simulink model "Lombardini_dual_fuel"  (R2024b)
settings: Solver=FixedStepAuto  StartTime=0.0  StopTime=2000  RelTol=1e-3  EnableMultiTasking=on
PreLoadFcn:
  | try, eval([bdroot '_setup']); catch, eval('model_setup', ''); end
InitFcn:
  | try, eval([bdroot '_setup']); catch, eval('model_setup', ''); end
model workspace (MAT data in the model file):
  PID_rpm = [1000 2000 3000 4000]
undefined symbols (not defined in the file): ECU555, motohawk_build_version, motohawk_get_target_image, motohawk_target_type, motohawk_trunc_name, motohawk_vardec_path
libraries: MotoHawk_lib x118, motohawk_annotations_lib x23, dspstat3 x13, motohawk_examples_lib x1, MotoHawk_Protocols_lib x1
(part 2 of 5)

== system Lombardini_dual_fuel/Background ==
  FMU : Inport
  f : TriggerPort  TriggerType=function-call  VariantControl=Variant
  Plant : Subsystem  mask(Display Image File){image_file='engine.jpg'}
      mask prompts: image_file "Image File"
      mask help:
      | Enter an image file on the current MATLAB path to display on this block.
      |
      | Double-clicking this block opens the contents of the subsystem.  Right-click and select 'Mask parameters...' to select a new image file.
      |
      | To use just the mask of this block in a model, but supply your own contents, break the link to the library.
      mask init:
      | try,
      | 	img = imread(image_file);
      | 	motohawk_block_image(gcb, image_file);
      | catch,
      | 	img = imread('image_not_found.jpg');
      | end
      settings: OpenFcn=open_system(gcb,'force')  MoveFcn=motohawk_block_image(gcb, motohawk_get_param_ws(gcb, 'image_file'));
      mask Display: image(img);
  motohawk_TitleBlock : motohawk_annotations_lib/motohawk_TitleBlock  BlockType_='Mototron_Title_Block'  ttl=[strrep(get_param(bdroot, 'Description') , '_', '\_') '\newline\rm' get_param(gcs, 'Name')]  copyright="'THE INFORMATION CONTAINED IN THIS\\newlineDRAWING IS THE SOLE PROPERTY OF\\newlineWOODWARD.  ANY REPRODUCTION IN\\newline PART OR AS A WHOLE WITHOUT THE\\newlineWRITTEN PERMISSION OF WOODWARD\\newline IS PROHIBITED.\\fontsize{16}\\rm\\copyright\\rm\\fontsize{10} 2017'"  address='\fontsize{22}\it\fontname{Arial Black}Woodward \fontname{Arial}\fontsize{10}\newline1081 Woodward Way, Fort Collins, CO, 80524\newlinemcs.woodward.com'  image_file='mh.jpg'  pretty_print=on  edit_text=[strrep(get_param(bdroot, 'Description') , '_', '\_') '\newline\rm' get_param(gcs, 'Name')]  edit_as=5
      settings: SourceProductName=MotoHawk Annotations
  motohawk_code_coverage : MotoHawk_lib/Extra Development Blocks/motohawk_code_coverage
      settings: SourceProductName=MotoHawk
  wires:
  FMU/1 -> Plant/1(FMU)

== system Lombardini_dual_fuel/Foreground ==
  FMU : Inport
  f : TriggerPort  TriggerType=function-call  VariantControl=Variant
  Controller : Subsystem  mask(Display Image File){image_file=motohawk_get_target_image(motohawk_target_type(bdroot))}
      mask prompts: image_file "Image File"
      mask help:
      | Enter an image file on the current MATLAB path to display on this block.
      |
      | Double-clicking this block opens the contents of the subsystem.  Right-click and select 'Mask parameters...' to select a new image file.
      |
      | To use just the mask of this block in a model, but supply your own contents, break the link to the library.
      mask init:
      | try,
      | 	img = imread(image_file);
      | 	motohawk_block_image(gcb, image_file);
      | catch,
      | 	img = imread('image_not_found.jpg');
      | end
      settings: OpenFcn=open_system(gcb,'force')  MoveFcn=motohawk_block_image(gcb, motohawk_get_param_ws(gcb, 'image_file'));
      mask Display: image(img);
  Plant : Subsystem  mask(Display Image File){image_file='engine.jpg'}
      mask prompts: image_file "Image File"
      mask help:
      | Enter an image file on the current MATLAB path to display on this block.
      |
      | Double-clicking this block opens the contents of the subsystem.  Right-click and select 'Mask parameters...' to select a new image file.
      |
      | To use just the mask of this block in a model, but supply your own contents, break the link to the library.
      mask init:
      | try,
      | 	img = imread(image_file);
      | 	motohawk_block_image(gcb, image_file);
      | catch,
      | 	img = imread('image_not_found.jpg');
      | end
      settings: OpenFcn=open_system(gcb,'force')  MoveFcn=motohawk_block_image(gcb, motohawk_get_param_ws(gcb, 'image_file'));
      mask Display: image(img);
  motohawk_TitleBlock : motohawk_annotations_lib/motohawk_TitleBlock  BlockType_='Mototron_Title_Block'  ttl=[strrep(get_param(bdroot, 'Description') , '_', '\_') '\newline\rm' get_param(gcs, 'Name')]  copyright="'THE INFORMATION CONTAINED IN THIS\\newlineDRAWING IS THE SOLE PROPERTY OF\\newlineWOODWARD.  ANY REPRODUCTION IN\\newline PART OR AS A WHOLE WITHOUT THE\\newlineWRITTEN PERMISSION OF WOODWARD\\newline IS PROHIBITED.\\fontsize{16}\\rm\\copyright\\rm\\fontsize{10} 2017'"  address='\fontsize{22}\it\fontname{Arial Black}Woodward \fontname{Arial}\fontsize{10}\newline1081 Woodward Way, Fort Collins, CO, 80524\newlinemcs.woodward.com'  image_file='mh.jpg'  pretty_print=on  edit_text=[strrep(get_param(bdroot, 'Description') , '_', '\_') '\newline\rm' get_param(gcs, 'Name')]  edit_as=5
      settings: SourceProductName=MotoHawk Annotations
  motohawk_code_coverage : MotoHawk_lib/Extra Development Blocks/motohawk_code_coverage
      settings: SourceProductName=MotoHawk
  Out1 : Outport
  wires:
  Plant/1(SensorBus) -> Controller/1(Sensors)
  Controller/1(Actuators) -> Out1/1, Plant/1(ActuatorBus)
  FMU/1 -> Plant/2(FMU)

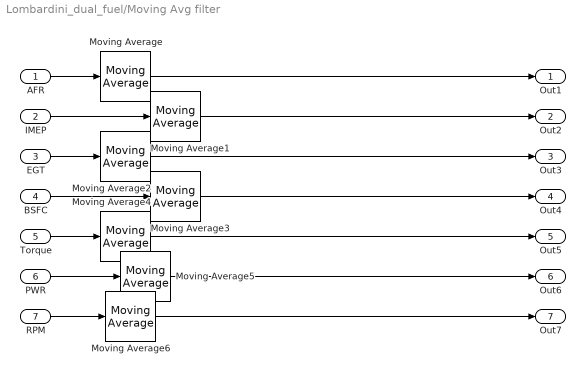
== system Lombardini_dual_fuel/Moving Avg filter ==
  AFR : Inport
  IMEP : Inport  Port=2
  EGT : Inport  Port=3
  BSFC : Inport  Port=4
  Torque : Inport  Port=5
  PWR : Inport  Port=6
  RPM : Inport  Port=7
  Moving Average : dspstat3/Moving Average  Method=Sliding window  ForgettingFactorPort=off  SpecifyWindowLength=on  WindowLength=200  OverlapLength=199  AllowArbitraryInputLength=off  ForgettingFactor=0.9  SimulateUsing=Interpreted execution
  Moving Average{1..6} (6 alike) : dspstat3/Moving Average  Method=Sliding window  ForgettingFactorPort=off  SpecifyWindowLength=on  WindowLength=100  OverlapLength=99  AllowArbitraryInputLength=off  ForgettingFactor=0.9  SimulateUsing=Interpreted execution
  Out1 : Outport
  Out2 : Outport  Port=2
  Out3 : Outport  Port=3
  Out4 : Outport  Port=4
  Out5 : Outport  Port=5
  Out6 : Outport  Port=6
  Out7 : Outport  Port=7
  wires:
  AFR/1 -> Moving Average/1
  RPM/1 -> Moving Average6/1
  IMEP/1 -> Moving Average1/1
  Moving Average1/1 -> Out2/1
  Moving Average2/1 -> Out3/1
  Moving Average5/1 -> Out6/1
  Moving Average/1 -> Out1/1
  BSFC/1 -> Moving Average3/1
  Moving Average4/1 -> Out5/1
  Torque/1 -> Moving Average4/1
  PWR/1 -> Moving Average5/1
  Moving Average3/1 -> Out4/1
  EGT/1 -> Moving Average2/1
  Moving Average6/1 -> Out7/1

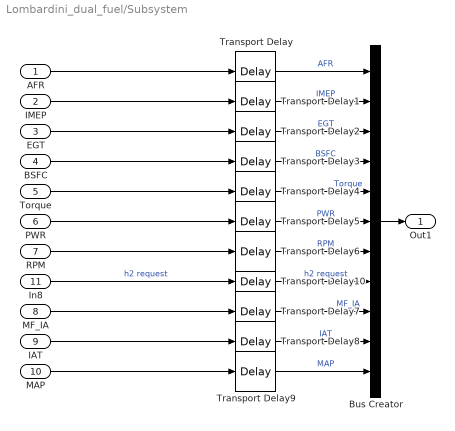
== system Lombardini_dual_fuel/Subsystem ==
  AFR : Inport
  IMEP : Inport  Port=2
  EGT : Inport  Port=3
  BSFC : Inport  Port=4
  Torque : Inport  Port=5
  PWR : Inport  Port=6
  RPM : Inport  Port=7
  MF_IA : Inport  Port=8
  IAT : Inport  Port=9
  MAP : Inport  Port=10
  In8 : Inport  Port=11
  Bus Creator : BusCreator  Inputs=11
  Transport Delay{,1..10} (11 alike) : TransportDelay  DelayTime=0.1
  Out1 : Outport
  wires:
  Transport Delay6/1 -> Bus Creator/7  "RPM"
  Transport Delay1/1 -> Bus Creator/2  "IMEP"
  Transport Delay5/1 -> Bus Creator/6  "PWR"
  Transport Delay2/1 -> Bus Creator/3  "EGT"
  AFR/1 -> Transport Delay/1
  Transport Delay/1 -> Bus Creator/1  "AFR"
  Transport Delay3/1 -> Bus Creator/4  "BSFC"
  Transport Delay4/1 -> Bus Creator/5  "Torque"
  RPM/1 -> Transport Delay6/1
  IMEP/1 -> Transport Delay1/1
  EGT/1 -> Transport Delay2/1
  PWR/1 -> Transport Delay5/1
  Bus Creator/1 -> Out1/1
  Torque/1 -> Transport Delay4/1
  BSFC/1 -> Transport Delay3/1
  In8/1 -> Transport Delay10/1  "h2 request"
  MF_IA/1 -> Transport Delay7/1
  Transport Delay7/1 -> Bus Creator/9  "MF_IA"
  MAP/1 -> Transport Delay9/1
  IAT/1 -> Transport Delay8/1
  Transport Delay8/1 -> Bus Creator/10  "IAT"
  Transport Delay9/1 -> Bus Creator/11  "MAP"
  Transport Delay10/1 -> Bus Creator/8  "h2 request"

== system Lombardini_dual_fuel/Subsystem1 ==
  In1 : Inport
  In3 : Inport  Port=2
  Moving Average1 : dspstat3/Moving Average  Method=Sliding window  ForgettingFactorPort=off  SpecifyWindowLength=on  WindowLength=100  OverlapLength=99  AllowArbitraryInputLength=off  ForgettingFactor=0.9  SimulateUsing=Interpreted execution
  Moving Average4 : dspstat3/Moving Average  Method=Sliding window  ForgettingFactorPort=off  SpecifyWindowLength=on  WindowLength=100  OverlapLength=99  AllowArbitraryInputLength=off  ForgettingFactor=0.9  SimulateUsing=Interpreted execution
  fuel energy : Outport
  imep gas exchange : Outport  Port=2
  wires:
  Moving Average1/1 -> imep gas exchange/1  "imep gas exchange"
  In1/1 -> Moving Average4/1
  In3/1 -> Moving Average1/1
  Moving Average4/1 -> fuel energy/1  "fuel energy"

== system Lombardini_dual_fuel/Background/Plant ==
  FMU : Inport
  Sensors : Subsystem
  motohawk_TitleBlock : motohawk_annotations_lib/motohawk_TitleBlock  BlockType_='Mototron_Title_Block'  ttl=[get_param(bdroot, 'Description') '\rm\newlineRead H/W sensors and Drive H/W actuators\newlineThe Sensors and Actuators busses should contain signals in engineering units\newline']  copyright="'THE INFORMATION CONTAINED IN THIS\\newlineDRAWING IS THE SOLE PROPERTY OF\\newlineWOODWARD.  ANY REPRODUCTION IN\\newline PART OR AS A WHOLE WITHOUT THE\\newlineWRITTEN PERMISSION OF WOODWARD\\newline IS PROHIBITED.\\fontsize{16}\\rm\\copyright\\rm\\fontsize{10} 2017'"  address='\fontsize{22}\it\fontname{Arial Black}Woodward \fontname{Arial}\fontsize{10}\newline1081 Woodward Way, Fort Collins, CO, 80524\newlinemcs.woodward.com'  image_file='mh.jpg'  pretty_print=on  edit_text=|  edit_as=6
      | [get_param(bdroot, 'Description') '\rm
      | 
      | 
      | Read H/W sensors and Drive H/W actuators
      | 
      | 
      | The Sensors and Actuators busses should contain signals in engineering units
      | 
      | 
      | ']
      settings: SourceProductName=MotoHawk Annotations
  wires:
  FMU/1 -> Sensors/1(In1)

== system Lombardini_dual_fuel/Foreground/Controller ==
  Sensors : Inport
  Calibration : Subsystem
  Characterization : Subsystem
  Controller : Subsystem
  Virtual Sensors : Subsystem
  motohawk_TitleBlock : motohawk_annotations_lib/motohawk_TitleBlock  BlockType_='Mototron_Title_Block'  ttl=[get_param(bdroot, 'Description') '\rm\newlineTop-level design of Controller\newlineVirtual Sensors model signals that are not available as H/W sensors\newlineCharacterization converts or linearizes Controller units to actuator units\newline']  copyright="'THE INFORMATION CONTAINED IN THIS\\newlineDRAWING IS THE SOLE PROPERTY OF\\newlineWOODWARD.  ANY REPRODUCTION IN\\newline PART OR AS A WHOLE WITHOUT THE\\newlineWRITTEN PERMISSION OF WOODWARD\\newline IS PROHIBITED.\\fontsize{16}\\rm\\copyright\\rm\\fontsize{10} 2017'"  address='\fontsize{22}\it\fontname{Arial Black}Woodward \fontname{Arial}\fontsize{10}\newline1081 Woodward Way, Fort Collins, CO, 80524\newlinemcs.woodward.com'  image_file='mh.jpg'  pretty_print=on  edit_text=|  edit_as=6
      | [get_param(bdroot, 'Description') '\rm
      | 
      | 
      | Top-level design of Controller
      | 
      | 
      | Virtual Sensors model signals that are not available as H/W sensors
      | 
      | 
      | Characterization converts or linearizes Controller units to actuator units
      | 
      | 
      | ']
      settings: SourceProductName=MotoHawk Annotations
  Actuators : Outport  VectorParamsAs1DForOutWhenUnconnected=off
  wires:
  Controller/1(Actuators) -> Characterization/1(Control)
  Virtual Sensors/1(Synth) -> Calibration/1(Sensor data), Controller/1(Sensors)
  Sensors/1 -> Virtual Sensors/1(Real)
  Characterization/1(Actuators) -> Actuators/1
  Calibration/1(Calibration data) -> Controller/2(Calibration)

== system Lombardini_dual_fuel/Foreground/Plant ==
  ActuatorBus : Inport
  FMU : Inport  Port=2
  Actuators : Subsystem
  Sensors : Subsystem
  motohawk_TitleBlock : motohawk_annotations_lib/motohawk_TitleBlock  BlockType_='Mototron_Title_Block'  ttl=[get_param(bdroot, 'Description') '\rm\newlineRead H/W sensors and Drive H/W actuators\newlineThe Sensors and Actuators busses should contain signals in engineering units\newline']  copyright="'THE INFORMATION CONTAINED IN THIS\\newlineDRAWING IS THE SOLE PROPERTY OF\\newlineWOODWARD.  ANY REPRODUCTION IN\\newline PART OR AS A WHOLE WITHOUT THE\\newlineWRITTEN PERMISSION OF WOODWARD\\newline IS PROHIBITED.\\fontsize{16}\\rm\\copyright\\rm\\fontsize{10} 2017'"  address='\fontsize{22}\it\fontname{Arial Black}Woodward \fontname{Arial}\fontsize{10}\newline1081 Woodward Way, Fort Collins, CO, 80524\newlinemcs.woodward.com'  image_file='mh.jpg'  pretty_print=on  edit_text=|  edit_as=6
      | [get_param(bdroot, 'Description') '\rm
      | 
      | 
      | Read H/W sensors and Drive H/W actuators
      | 
      | 
      | The Sensors and Actuators busses should contain signals in engineering units
      | 
      | 
      | ']
      settings: SourceProductName=MotoHawk Annotations
  SensorBus : Outport  VectorParamsAs1DForOutWhenUnconnected=off
  wires:
  Sensors/1(Sensors) -> SensorBus/1
  ActuatorBus/1 -> Actuators/1(Actuators)
  FMU/1 -> Sensors/1(In1)

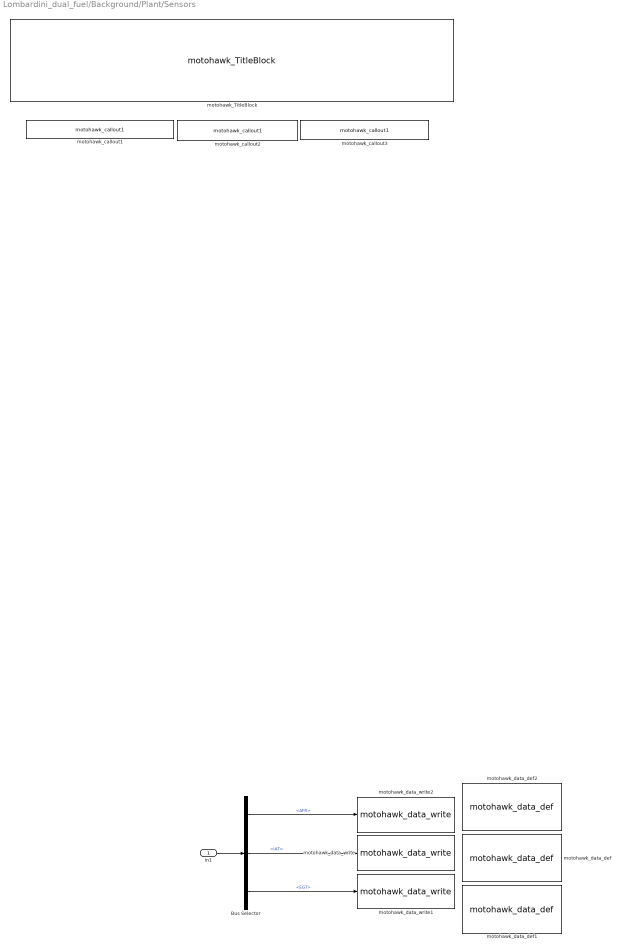
== system Lombardini_dual_fuel/Background/Plant/Sensors ==
  In1 : Inport
  Bus Selector : BusSelector  OutputSignals=AFR,IAT,EGT
  motohawk_TitleBlock : motohawk_annotations_lib/motohawk_TitleBlock  BlockType_='Mototron_Title_Block'  ttl=[get_param(bdroot, 'Description') '\rm\newlineSample H/W sensors, such as:\newlineA/D converters, digital inputs, frequency inputs, and engine encoder\newline']  copyright="'THE INFORMATION CONTAINED IN THIS\\newlineDRAWING IS THE SOLE PROPERTY OF\\newlineWOODWARD.  ANY REPRODUCTION IN\\newline PART OR AS A WHOLE WITHOUT THE\\newlineWRITTEN PERMISSION OF WOODWARD\\newline IS PROHIBITED.\\fontsize{16}\\rm\\copyright\\rm\\fontsize{10} 2017'"  address='\fontsize{22}\it\fontname{Arial Black}Woodward \fontname{Arial}\fontsize{10}\newline1081 Woodward Way, Fort Collins, CO, 80524\newlinemcs.woodward.com'  image_file='mh.jpg'  pretty_print=on  edit_text=|  edit_as=6
      | [get_param(bdroot, 'Description') '\rm
      | 
      | 
      | Sample H/W sensors, such as:
      | 
      | 
      | A/D converters, digital inputs, frequency inputs, and engine encoder
      | 
      | 
      | ']
      settings: SourceProductName=MotoHawk Annotations
  motohawk_callout1 : motohawk_annotations_lib/motohawk_callout1  BlockType_='Mototron_harea'  desc='Read from H/W'  edit_text=Read from H/W  edit_as=0
      settings: SourceProductName=MotoHawk Annotations
  motohawk_callout2 : motohawk_annotations_lib/motohawk_callout1  BlockType_='Mototron_harea'  desc='Convert to Engineering Units'  edit_text=Convert to Engineering Units  edit_as=0
      settings: SourceProductName=MotoHawk Annotations
  motohawk_callout3 : motohawk_annotations_lib/motohawk_callout1  BlockType_='Mototron_harea'  desc='Create a Bus of Sensors'  edit_text=Create a Bus of Sensors  edit_as=0
      settings: SourceProductName=MotoHawk Annotations
  motohawk_data_def : MotoHawk_lib/Data Storage Blocks/motohawk_data_def  nam='IAT_slow'  container_nam=''  data=5  typ=double  struct_nam='MyStruct'  storage=Volatile  outputRef=off  mem_region_use=off  mem_region_name='SERIAL_EE'  use_vardec=on  window=Display  ovr_cals=on  read_level=1  write_level=1  view_as=Number  enum_struct={'Disabled', 'Enabled'}  vector_style=Wide Row  row_header_enum=''  col_header_enum=''  mototune_group=motohawk_vardec_path(gcb)  help=''  units=''  min_val=-inf  max_val=inf  precision=''  gain=1  offset=0  exp=1  use_help_units=off  use_header_enum=off  use_min_max=off  use_precision=off  use_mototune_group=off  eval_name=MyData  struct_instances=motohawk_sfun_data_def_struct_instances  vardecs=motohawk_sfun_data_def_vardecs  data_stores=motohawk_sfun_data_def_data_stores
      settings: SourceProductName=MotoHawk
  motohawk_data_def1 : MotoHawk_lib/Data Storage Blocks/motohawk_data_def  nam='EGT_100ms'  container_nam=''  data=5  typ=double  struct_nam='MyStruct'  storage=Volatile  outputRef=off  mem_region_use=off  mem_region_name='SERIAL_EE'  use_vardec=on  window=Display  ovr_cals=on  read_level=1  write_level=1  view_as=Number  enum_struct={'Disabled', 'Enabled'}  vector_style=Wide Row  row_header_enum=''  col_header_enum=''  mototune_group=motohawk_vardec_path(gcb)  help=''  units=''  min_val=-inf  max_val=inf  precision=''  gain=1  offset=0  exp=1  use_help_units=off  use_header_enum=off  use_min_max=off  use_precision=off  use_mototune_group=off  eval_name=MyData  struct_instances=motohawk_sfun_data_def_struct_instances  vardecs=motohawk_sfun_data_def_vardecs  data_stores=motohawk_sfun_data_def_data_stores
      settings: SourceProductName=MotoHawk
  motohawk_data_def2 : MotoHawk_lib/Data Storage Blocks/motohawk_data_def  nam='AFR_100ms'  container_nam=''  data=5  typ=double  struct_nam='MyStruct'  storage=Volatile  outputRef=off  mem_region_use=off  mem_region_name='SERIAL_EE'  use_vardec=on  window=Display  ovr_cals=on  read_level=1  write_level=1  view_as=Number  enum_struct={'Disabled', 'Enabled'}  vector_style=Wide Row  row_header_enum=''  col_header_enum=''  mototune_group=motohawk_vardec_path(gcb)  help=''  units=''  min_val=-inf  max_val=inf  precision=''  gain=1  offset=0  exp=1  use_help_units=off  use_header_enum=off  use_min_max=off  use_precision=off  use_mototune_group=off  eval_name=MyData  struct_instances=motohawk_sfun_data_def_struct_instances  vardecs=motohawk_sfun_data_def_vardecs  data_stores=motohawk_sfun_data_def_data_stores
      settings: SourceProductName=MotoHawk
  motohawk_data_write : MotoHawk_lib/Data Storage Blocks/motohawk_data_write  source=Lookup By Name  structure=Scalar  operation=Write entire data structure at once  sz_vec=9  sz_row=2  sz_col=9  use_access_prot=off  use_access_prot_status=off  typ=double  nam='IAT_slow'  checkNull=on  write_read_only=off  struct_inst_name=''  struct_name='MyStruct'
      settings: SourceProductName=MotoHawk
  motohawk_data_write1 : MotoHawk_lib/Data Storage Blocks/motohawk_data_write  source=Lookup By Name  structure=Scalar  operation=Write entire data structure at once  sz_vec=9  sz_row=2  sz_col=9  use_access_prot=off  use_access_prot_status=off  typ=double  nam='EGT_100ms'  checkNull=on  write_read_only=off  struct_inst_name=''  struct_name='MyStruct'
      settings: SourceProductName=MotoHawk
  motohawk_data_write2 : MotoHawk_lib/Data Storage Blocks/motohawk_data_write  source=Lookup By Name  structure=Scalar  operation=Write entire data structure at once  sz_vec=9  sz_row=2  sz_col=9  use_access_prot=off  use_access_prot_status=off  typ=double  nam='AFR_100ms'  checkNull=on  write_read_only=off  struct_inst_name=''  struct_name='MyStruct'
      settings: SourceProductName=MotoHawk
  wires:
  Bus Selector/3 -> motohawk_data_write1/1  "<EGT>"
  In1/1 -> Bus Selector/1
  Bus Selector/2 -> motohawk_data_write/1  "<IAT>"
  Bus Selector/1 -> motohawk_data_write2/1  "<AFR>"

== system Lombardini_dual_fuel/Foreground/Controller/Calibration ==
  Sensor data : Inport
  Bus Creator : BusCreator  Inputs=1
  Bus Selector : BusSelector  OutputSignals=RPM,MAP,U_Bat,Load,IAT,P_CR
  Calibration parameters : Subsystem
  motohawk_TitleBlock : motohawk_annotations_lib/motohawk_TitleBlock  BlockType_='Mototron_Title_Block'  ttl=[get_param(bdroot, 'Description') '\newline\rmVirtual Sensors\newlineModel signals that are not available as H/W sensors,\newlinebut that would be used by the controller if they were physically available']  copyright="'THE INFORMATION CONTAINED IN THIS\\newlineDRAWING IS THE SOLE PROPERTY OF\\newlineWOODWARD.  ANY REPRODUCTION IN\\newline PART OR AS A WHOLE WITHOUT THE\\newlineWRITTEN PERMISSION OF WOODWARD\\newline IS PROHIBITED.\\fontsize{16}\\rm\\copyright\\rm\\fontsize{10} 2017'"  address='\fontsize{22}\it\fontname{Arial Black}Woodward \fontname{Arial}\fontsize{10}\newline1081 Woodward Way, Fort Collins, CO, 80524\newlinemcs.woodward.com'  image_file='mh.jpg'  pretty_print=on  edit_text="strrep([get_param(bdroot, 'Description')  '\\rm\\newline'  get_param(gcs, 'Name')], '_', '\\_')"  edit_as=255
      settings: SourceProductName=MotoHawk Annotations
  Calibration data : Outport  VectorParamsAs1DForOutWhenUnconnected=off
  wires:
  Bus Creator/1 -> Calibration data/1
  Sensor data/1 -> Bus Selector/1
  Bus Selector/1 -> Calibration parameters/1(RPM)  "<RPM>"
  Bus Selector/2 -> Calibration parameters/2(MAP)  "<MAP>"
  Bus Selector/3 -> Calibration parameters/3(U_bat)  "<U_Bat>"
  Bus Selector/4 -> Calibration parameters/4(Load)  "<Load>"
  Bus Selector/5 -> Calibration parameters/5(IAT)  "<IAT>"
  Bus Selector/6 -> Calibration parameters/6(P_CR)  "<P_CR>"
  Calibration parameters/1(Calibration) -> Bus Creator/1

== system Lombardini_dual_fuel/Foreground/Controller/Characterization ==
  note: - Outputs from here are still entirely in engineering\newlineunits, but are converted from a form used by the\newlinecontroller to one required by the physical actuators
  note: - This is a good place to put a PID controller that\newlineis always enabled, such as an electronic throttle\newlinecontroller (ETC)\newline\newline- The controller outputs a desired setpoint,\newlinea block in this subsystem performs the\newlineclosed-loop control to that position.
  note: \fontsize{16}\bfTo Do:\newlineConvert from desired controller units\newlineto those required by each actuator.
  note: \fontsize{16}\bfTo Do:\newlinePass-through actuators\newlinethat do not require modification.
  Control : Inport
  Bus Creator : BusCreator  Inputs=5
  Bus Selector : BusSelector  OutputSignals=InjM_D,inj_H2,P_CR_Res
  Bus Selector2 : BusSelector  OutputSignals=SOI,Inj_Duration
  Data Type Conversion : DataTypeConversion
  Data Type Conversion1 : DataTypeConversion
  Data Type Conversion2 : DataTypeConversion
  motohawk_TitleBlock : motohawk_annotations_lib/motohawk_TitleBlock  BlockType_='Mototron_Title_Block'  ttl=[get_param(bdroot, 'Description') '\rm\newlineActuator Characterization\newlineConverts or linearizes controller units to actuator units\newline']  copyright="'THE INFORMATION CONTAINED IN THIS\\newlineDRAWING IS THE SOLE PROPERTY OF\\newlineWOODWARD.  ANY REPRODUCTION IN\\newline PART OR AS A WHOLE WITHOUT THE\\newlineWRITTEN PERMISSION OF WOODWARD\\newline IS PROHIBITED.\\fontsize{16}\\rm\\copyright\\rm\\fontsize{10} 2017'"  address='\fontsize{22}\it\fontname{Arial Black}Woodward \fontname{Arial}\fontsize{10}\newline1081 Woodward Way, Fort Collins, CO, 80524\newlinemcs.woodward.com'  image_file='mh.jpg'  pretty_print=on  edit_text=|  edit_as=6
      | [get_param(bdroot, 'Description') '\rm
      | 
      | 
      | Actuator Characterization
      | 
      | 
      | Converts or linearizes controller units to actuator units
      | 
      | 
      | ']
      settings: SourceProductName=MotoHawk Annotations
  Actuators : Outport  VectorParamsAs1DForOutWhenUnconnected=off
  wires:
  Bus Creator/1 -> Actuators/1
  Bus Selector2/1 -> Data Type Conversion/1  "<SOI>"
  Control/1 -> Bus Selector2/1, Bus Selector/1
  Data Type Conversion/1 -> Bus Creator/4  "FuelStartAngle"
  Data Type Conversion1/1 -> Bus Creator/5  "FuelStopDuration"
  Bus Selector/1 -> Bus Creator/1  "<InjM_D>"
  Bus Selector2/2 -> Data Type Conversion1/1  "<Inj_Duration>"
  Bus Selector/3 -> Data Type Conversion2/1  "<P_CR_Res>"
  Data Type Conversion2/1 -> Bus Creator/3  "P_CR_Res"
  Bus Selector/2 -> Bus Creator/2  "<inj_H2>"

== system Lombardini_dual_fuel/Foreground/Controller/Controller ==
  note: Simplify as much as possible, by offloading work to the\newlineVirtual Sensors and Actuator Characterization subsystems
  note: If the controller contains multiple states,\newlinecreate a StateFlow representation of the state machine here.
  note: \fontsize{16}\bfTo Do:\newlinePerform the actions required by the controller.
  Sensors : Inport
  Calibration : Inport  Port=2
  Bus Creator : BusCreator  Inputs=5
  Bus Selector : BusSelector  OutputSignals=RPM,MAP,AFR,IAT,Load,P_CR,h2 request
  CR Pressure control : Subsystem
  Fuel control : Subsystem
  motohawk_TitleBlock : motohawk_annotations_lib/motohawk_TitleBlock  BlockType_='Mototron_Title_Block'  ttl=[get_param(bdroot, 'Description') '\rm\newlineEngine control system\newlineConsists of simple tables for spark and fuel\newline']  copyright="'THE INFORMATION CONTAINED IN THIS\\newlineDRAWING IS THE SOLE PROPERTY OF\\newlineWOODWARD.  ANY REPRODUCTION IN\\newline PART OR AS A WHOLE WITHOUT THE\\newlineWRITTEN PERMISSION OF WOODWARD\\newline IS PROHIBITED.\\fontsize{16}\\rm\\copyright\\rm\\fontsize{10} 2017'"  address='\fontsize{22}\it\fontname{Arial Black}Woodward \fontname{Arial}\fontsize{10}\newline1081 Woodward Way, Fort Collins, CO, 80524\newlinemcs.woodward.com'  image_file='mh.jpg'  pretty_print=on  edit_text=|  edit_as=6
      | [get_param(bdroot, 'Description') '\rm
      | 
      | 
      | Engine control system
      | 
      | 
      | Consists of simple tables for spark and fuel
      | 
      | 
      | ']
      settings: SourceProductName=MotoHawk Annotations
  motohawk_data_read : MotoHawk_lib/Data Storage Blocks/motohawk_data_read  source=Lookup By Name  structure=Scalar  operation=Read scalar from location by index  sz_vec=4  sz_row=2  sz_col=3  use_access_prot=off  use_access_prot_status=off  typ=double  nam='IAT_slow'  checkNull=on  struct_inst_name='MyData'  struct_nam='MyStruct'
      settings: SourceProductName=MotoHawk
  motohawk_data_read1 : MotoHawk_lib/Data Storage Blocks/motohawk_data_read  source=Lookup By Name  structure=Scalar  operation=Read scalar from location by index  sz_vec=4  sz_row=2  sz_col=3  use_access_prot=off  use_access_prot_status=off  typ=double  nam='EGT_100ms'  checkNull=on  struct_inst_name='MyData'  struct_nam='MyStruct'
      settings: SourceProductName=MotoHawk
  motohawk_data_read2 : MotoHawk_lib/Data Storage Blocks/motohawk_data_read  source=Lookup By Name  structure=Scalar  operation=Read scalar from location by index  sz_vec=4  sz_row=2  sz_col=3  use_access_prot=off  use_access_prot_status=off  typ=double  nam='AFR_100ms'  checkNull=on  struct_inst_name='MyData'  struct_nam='MyStruct'
      settings: SourceProductName=MotoHawk
  Actuators : Outport  VectorParamsAs1DForOutWhenUnconnected=off
  wires:
  Sensors/1 -> Bus Selector/1
  Bus Selector/5 -> CR Pressure control/1(Load)  "<Load>"
  Bus Selector/3 -> Fuel control/3(AFR_Ref)  "<AFR>"
  Bus Creator/1 -> Actuators/1
  Bus Selector/2 -> Fuel control/2(MAP)  "<MAP>"
  Bus Selector/6 -> CR Pressure control/3(<P_CR>)  "<P_CR>"
  Bus Selector/1 -> CR Pressure control/2(RPM), Fuel control/1(RPM)  "<RPM>"
  Fuel control/1(InjM_D) -> Bus Creator/1  "InjM_D"
  Fuel control/2(SOI) -> Bus Creator/2  "SOI"
  Fuel control/3(Inj_Duration) -> Bus Creator/3  "Inj_Duration"
  CR Pressure control/1(P_CR_Res) -> Bus Creator/5  "P_CR_Res"
  Bus Selector/7 -> Fuel control/5(Energy fraction)  "<h2 request>"
  Fuel control/4(InjM_H2) -> Bus Creator/4  "inj_H2"
  Calibration/1 -> Fuel control/6(Calibration)
  motohawk_data_read/1 -> Fuel control/4(IAT)

== system Lombardini_dual_fuel/Foreground/Controller/Virtual Sensors ==
  Real : Inport
  Bus Creator : BusCreator  Inputs=13
  Bus Selector : BusSelector  OutputSignals=RPMInst,RPM,MAP,P_H2,T_H2,P_Baro,U_Bat,P_Fuel,Load,IAT,P_CR,signal12.AFR,signal12.h2 request
  motohawk_TitleBlock : motohawk_annotations_lib/motohawk_TitleBlock  BlockType_='Mototron_Title_Block'  ttl=[get_param(bdroot, 'Description') '\newline\rmVirtual Sensors\newlineModel signals that are not available as H/W sensors,\newlinebut that would be used by the controller if they were physically available']  copyright="'THE INFORMATION CONTAINED IN THIS\\newlineDRAWING IS THE SOLE PROPERTY OF\\newlineWOODWARD.  ANY REPRODUCTION IN\\newline PART OR AS A WHOLE WITHOUT THE\\newlineWRITTEN PERMISSION OF WOODWARD\\newline IS PROHIBITED.\\fontsize{16}\\rm\\copyright\\rm\\fontsize{10} 2017'"  address='\fontsize{22}\it\fontname{Arial Black}Woodward \fontname{Arial}\fontsize{10}\newline1081 Woodward Way, Fort Collins, CO, 80524\newlinemcs.woodward.com'  image_file='mh.jpg'  pretty_print=on  edit_text="strrep([get_param(bdroot, 'Description')  '\\rm\\newline'  get_param(gcs, 'Name')], '_', '\\_')"  edit_as=255
      settings: SourceProductName=MotoHawk Annotations
  Synth : Outport  VectorParamsAs1DForOutWhenUnconnected=off
  wires:
  Real/1 -> Bus Selector/1
  Bus Selector/1 -> Bus Creator/1  "<RPMInst>"
  Bus Selector/2 -> Bus Creator/2  "<RPM>"
  Bus Creator/1 -> Synth/1
  Bus Selector/3 -> Bus Creator/3  "<MAP>"
  Bus Selector/4 -> Bus Creator/4  "<P_H2>"
  Bus Selector/7 -> Bus Creator/7  "<U_Bat>"
  Bus Selector/8 -> Bus Creator/8  "<P_Fuel>"
  Bus Selector/5 -> Bus Creator/5  "<T_H2>"
  Bus Selector/6 -> Bus Creator/6  "<P_Baro>"
  Bus Selector/9 -> Bus Creator/9  "<Load>"
  Bus Selector/10 -> Bus Creator/10  "<IAT>"
  Bus Selector/11 -> Bus Creator/11  "<P_CR>"
  Bus Selector/12 -> Bus Creator/12  "<AFR>"
  Bus Selector/13 -> Bus Creator/13  "<h2 request>"

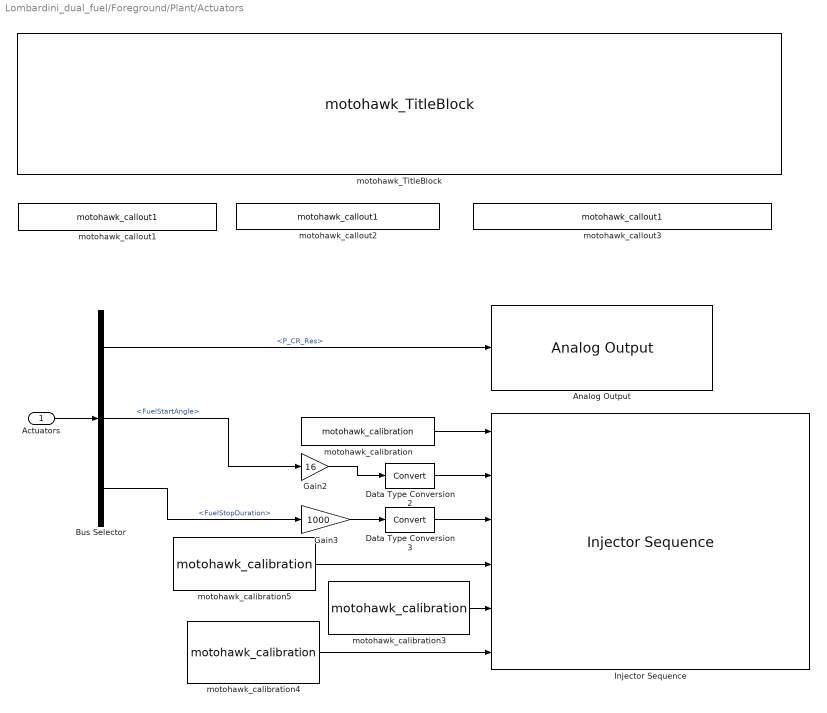
== system Lombardini_dual_fuel/Foreground/Plant/Actuators ==
  Actuators : Inport
  Analog Output : MotoHawk_lib/Analog I//O Blocks/Analog Output  res_name='P_CR_Res'  text_resource=(None)  code_resource=NONE  val_resource=-1  target=ECU555-48-0403  resource_enum_str=(None)=-1
      settings: SourceProductName=MotoHawk
  Bus Selector : BusSelector  OutputSignals=P_CR_Res,FuelStartAngle,FuelStopDuration
  Data Type Conversion2 : DataTypeConversion
  Data Type Conversion3 : DataTypeConversion
  Gain2 : Gain  Gain=16  SaturateOnIntegerOverflow=on  OutDataTypeStr=Inherit: Same as input  ParamDataTypeStr=Inherit: Same as input
  Gain3 : Gain  Gain=1000  SaturateOnIntegerOverflow=on  OutDataTypeStr=Inherit: Same as input  ParamDataTypeStr=Inherit: Same as input
  Injector Sequence : MotoHawk_lib/Advanced Digital I//O/Injector Sequence  text_resource=(None)  code_resource=NONE  val_resource=-1  target=ECU555-48-0403  resource_enum_str=(None)=-1,FUEL 1=12,FUEL 2=13,FUEL 3=14,FUEL 4=15  sequence_type=Standard (Injector per cylinder)  behavior=Standard  update_mode=OS  granularity=Fine  use_makeup=off  min_eoi_soi_angle=90  use_diag=off  show_trans_enable=off  min_duration_mode=Static  min_duration=1.5  use_vardec=off  nam='INJ_'  read_level=1  write_level=1  group='System | I/O Pins | Injector Config'
      settings: SourceProductName=MotoHawk
  motohawk_TitleBlock : motohawk_annotations_lib/motohawk_TitleBlock  BlockType_='Mototron_Title_Block'  ttl=[get_param(bdroot, 'Description') '\rm\newlineSample H/W sensors, such as:\newlineA/D converters, digital inputs, frequency inputs, and engine encoder\newline']  copyright="'THE INFORMATION CONTAINED IN THIS\\newlineDRAWING IS THE SOLE PROPERTY OF\\newlineWOODWARD.  ANY REPRODUCTION IN\\newline PART OR AS A WHOLE WITHOUT THE\\newlineWRITTEN PERMISSION OF WOODWARD\\newline IS PROHIBITED.\\fontsize{16}\\rm\\copyright\\rm\\fontsize{10} 2017'"  address='\fontsize{22}\it\fontname{Arial Black}Woodward \fontname{Arial}\fontsize{10}\newline1081 Woodward Way, Fort Collins, CO, 80524\newlinemcs.woodward.com'  image_file='mh.jpg'  pretty_print=on  edit_text=|  edit_as=6
      | [get_param(bdroot, 'Description') '\rm
      | 
      | 
      | Sample H/W sensors, such as:
      | 
      | 
      | A/D converters, digital inputs, frequency inputs, and engine encoder
      | 
      | 
      | ']
      settings: SourceProductName=MotoHawk Annotations
  motohawk_calibration : MotoHawk_lib/Calibration & Probing Blocks/motohawk_calibration  name_source=Use Parameter  nam='InjectorEnable'  val=false  storage=Display  ovr_cals=on  data_type=Inherit from 'Default Value'  mem_region_use=off  mem_region_name='SERIAL_EE'  read_level=1  write_level=1  view_as=Enumeration  enum_struct={'Disabled', 'Enabled'}  vector_style=Wide Row  row_header_enum={}  col_header_enum={}  mototune_group=motohawk_vardec_path(gcb)  help=''  units=''  min_val=-inf  max_val=inf  precision=''  gain=1  offset=0  exp=1  show_more=on  use_help_units=off  use_header_enum=off  use_min_max=off  use_precision=off  use_mototune_group=off  data_stores=motohawk_sfun_calibration_data_stores
      settings: SourceProductName=MotoHawk
  motohawk_calibration3 : MotoHawk_lib/Calibration & Probing Blocks/motohawk_calibration  name_source=Use Parameter  nam='InjectorMaxDuration'  val=500000  storage=Calibration  ovr_cals=on  data_type=Inherit via back propagation  mem_region_use=off  mem_region_name='SERIAL_EE'  read_level=1  write_level=1  view_as=Number  enum_struct={'Disabled', 'Enabled'}  vector_style=Wide Row  row_header_enum={}  col_header_enum={}  mototune_group=motohawk_vardec_path(gcb)  help="'Maximum duration for an injector pulse.  Must be a multiple of 5ms'"  units='us'  min_val=-inf  max_val=inf  precision=''  gain=1  offset=0  exp=1  show_more=on  use_help_units=on  use_header_enum=off  use_min_max=off  use_precision=off  use_mototune_group=off  data_stores=motohawk_sfun_calibration_data_stores
      settings: SourceProductName=MotoHawk
  motohawk_calibration4 : MotoHawk_lib/Calibration & Probing Blocks/motohawk_calibration  name_source=Use Parameter  nam='InjectorElectricalOffset'  val=0  storage=Calibration  ovr_cals=on  data_type=Inherit via back propagation  mem_region_use=off  mem_region_name='SERIAL_EE'  read_level=1  write_level=1  view_as=Number  enum_struct={'Disabled', 'Enabled'}  vector_style=Wide Row  row_header_enum={}  col_header_enum={}  mototune_group=motohawk_vardec_path(gcb)  help='Extra duration added to each generated pulse to account for the injector turn on and turn off time'  units='us'  min_val=-inf  max_val=inf  precision=''  gain=1  offset=0  exp=1  show_more=on  use_help_units=on  use_header_enum=off  use_min_max=off  use_precision=off  use_mototune_group=off  data_stores=motohawk_sfun_calibration_data_stores
      settings: SourceProductName=MotoHawk
  motohawk_calibration5 : MotoHawk_lib/Calibration & Probing Blocks/motohawk_calibration  name_source=Use Parameter  nam='InjectorPeakDuration'  val=0  storage=Calibration  ovr_cals=on  data_type=Inherit via back propagation  mem_region_use=off  mem_region_name='SERIAL_EE'  read_level=1  write_level=1  view_as=Number  enum_struct={'Disabled', 'Enabled'}  vector_style=Wide Row  row_header_enum={}  col_header_enum={}  mototune_group=motohawk_vardec_path(gcb)  help='For a low-impedance injector using the peak-and-hold driver, the duration of the peak portion of the total injector pulse'  units='us'  min_val=-inf  max_val=inf  precision=''  gain=1  offset=0  exp=1  show_more=on  use_help_units=on  use_header_enum=off  use_min_max=off  use_precision=off  use_mototune_group=off  data_stores=motohawk_sfun_calibration_data_stores
      settings: SourceProductName=MotoHawk
  motohawk_callout1 : motohawk_annotations_lib/motohawk_callout1  BlockType_='Mototron_harea'  desc='Read from Bus of Actuators'  edit_text=Read from Bus of Actuators  edit_as=0
      settings: SourceProductName=MotoHawk Annotations
  motohawk_callout2 : motohawk_annotations_lib/motohawk_callout1  BlockType_='Mototron_harea'  desc='Convert from Engineering Units'  edit_text=Convert from Engineering Units  edit_as=0
      settings: SourceProductName=MotoHawk Annotations
  motohawk_callout3 : motohawk_annotations_lib/motohawk_callout1  BlockType_='Mototron_harea'  desc='Drive H/W Actuators'  edit_text=Drive H/W Actuators  edit_as=0
      settings: SourceProductName=MotoHawk Annotations
  wires:
  Actuators/1 -> Bus Selector/1
  Gain3/1 -> Data Type Conversion3/1
  Gain2/1 -> Data Type Conversion2/1
  Bus Selector/2 -> Gain2/1  "<FuelStartAngle>"
  Bus Selector/3 -> Gain3/1  "<FuelStopDuration>"
  Data Type Conversion2/1 -> Injector Sequence/2
  Data Type Conversion3/1 -> Injector Sequence/3
  motohawk_calibration3/1 -> Injector Sequence/5
  motohawk_calibration4/1 -> Injector Sequence/6
  motohawk_calibration5/1 -> Injector Sequence/4
  motohawk_calibration/1 -> Injector Sequence/1
  Bus Selector/1 -> Analog Output/1  "<P_CR_Res>"

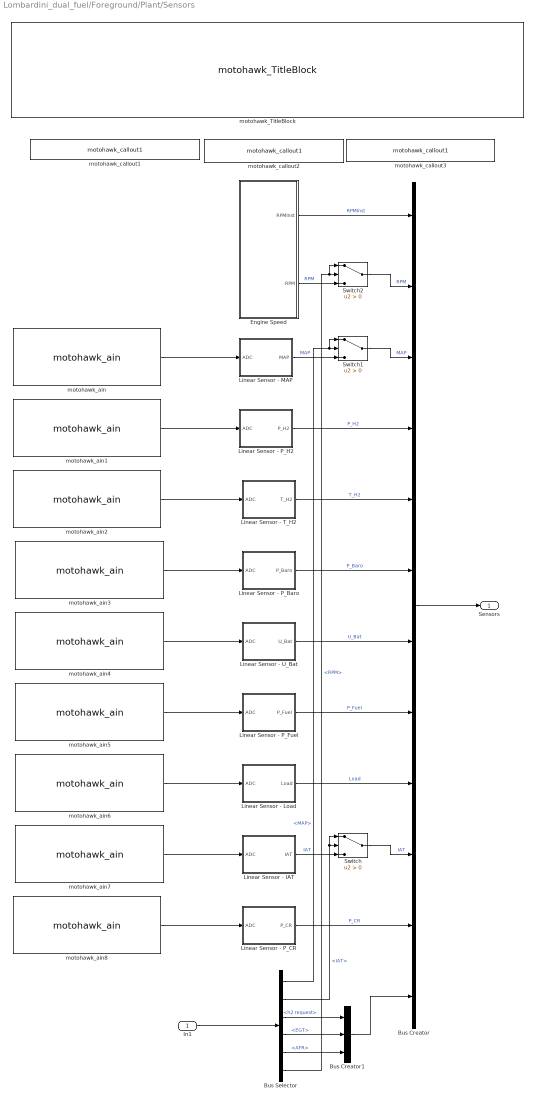
== system Lombardini_dual_fuel/Foreground/Plant/Sensors ==
  In1 : Inport
  Bus Creator : BusCreator  Inputs=12
  Bus Creator1 : BusCreator  Inputs=3
  Bus Selector : BusSelector  OutputSignals=MAP,IAT,h2 request,EGT,AFR,RPM
  Engine Speed : Subsystem
  Linear Sensor - IAT : Subsystem
  Linear Sensor - Load : Subsystem
  Linear Sensor - MAP : Subsystem
  Linear Sensor - P_Baro : Subsystem
  Linear Sensor - P_CR : Subsystem
  Linear Sensor - P_Fuel : Subsystem
  Linear Sensor - P_H2 : Subsystem
  Linear Sensor - T_H2 : Subsystem
  Linear Sensor - U_Bat : Subsystem
  Switch : Switch  Criteria=u2 > Threshold  SaturateOnIntegerOverflow=off  InputSameDT=off
  Switch1 : Switch  Criteria=u2 > Threshold  SaturateOnIntegerOverflow=off  InputSameDT=off
  Switch2 : Switch  Criteria=u2 > Threshold  SaturateOnIntegerOverflow=off  InputSameDT=off
  motohawk_TitleBlock : motohawk_annotations_lib/motohawk_TitleBlock  BlockType_='Mototron_Title_Block'  ttl=[get_param(bdroot, 'Description') '\rm\newlineSample H/W sensors, such as:\newlineA/D converters, digital inputs, frequency inputs, and engine encoder\newline']  copyright="'THE INFORMATION CONTAINED IN THIS\\newlineDRAWING IS THE SOLE PROPERTY OF\\newlineWOODWARD.  ANY REPRODUCTION IN\\newline PART OR AS A WHOLE WITHOUT THE\\newlineWRITTEN PERMISSION OF WOODWARD\\newline IS PROHIBITED.\\fontsize{16}\\rm\\copyright\\rm\\fontsize{10} 2017'"  address='\fontsize{22}\it\fontname{Arial Black}Woodward \fontname{Arial}\fontsize{10}\newline1081 Woodward Way, Fort Collins, CO, 80524\newlinemcs.woodward.com'  image_file='mh.jpg'  pretty_print=on  edit_text=|  edit_as=6
      | [get_param(bdroot, 'Description') '\rm
      | 
      | 
      | Sample H/W sensors, such as:
      | 
      | 
      | A/D converters, digital inputs, frequency inputs, and engine encoder
      | 
      | 
      | ']
      settings: SourceProductName=MotoHawk Annotations
  motohawk_ain : MotoHawk_lib/Analog I//O Blocks/motohawk_ain  res_name='MAP'  text_resource=AN1M  code_resource=NONE  val_resource=-1  target=ECU555-48-0403  resource_enum_str=(None)=-1,ECUP=53,DRVP=54,XDRP=55,AN1M=56,AN2M=57,AN3M=58,AN4M=59,AN5M=60,AN9M=64,AN10M=65,AN11M=66,AN14M=69,AN15M=70,AN18M=73,AN19M=74  altref=5V Reference  typ=uint16  num_adc_bits=10  use_stat=off  use_vardec=off  nam='RTD1_MW'  read_level=1  write_level=1  group='System | I/O Pins | Inputs Config'  use_altref=off  errorHandle=Ignore  errorHandleEdit='Warn'  altref_option_1=off  altref_option_2=off  altref_option_3=off  altref_option_4=off  altref_option_5=off  altref_option_6=off
      settings: SourceProductName=MotoHawk
  motohawk_ain1 : MotoHawk_lib/Analog I//O Blocks/motohawk_ain  res_name='P_H2'  text_resource=(None)  code_resource=NONE  val_resource=-1  target=ECU555-48-0403  resource_enum_str=(None)=-1,ECUP=53,DRVP=54,XDRP=55,AN1M=56,AN2M=57,AN3M=58,AN4M=59,AN5M=60,AN9M=64,AN10M=65,AN11M=66,AN14M=69,AN15M=70,AN18M=73,AN19M=74  altref=5V Reference  typ=uint16  num_adc_bits=12  use_stat=off  use_vardec=off  nam='RTD1_MW'  read_level=1  write_level=1  group='System | I/O Pins | Inputs Config'  use_altref=off  errorHandle=Ignore  errorHandleEdit='Warn'  altref_option_1=off  altref_option_2=off  altref_option_3=off  altref_option_4=off  altref_option_5=off  altref_option_6=off
      settings: SourceProductName=MotoHawk
  motohawk_ain2 : MotoHawk_lib/Analog I//O Blocks/motohawk_ain  res_name='T_H2'  text_resource=(None)  code_resource=NONE  val_resource=-1  target=ECU555-48-0403  resource_enum_str=(None)=-1,ECUP=53,DRVP=54,XDRP=55,AN1M=56,AN2M=57,AN3M=58,AN4M=59,AN5M=60,AN9M=64,AN10M=65,AN11M=66,AN14M=69,AN15M=70,AN18M=73,AN19M=74  altref=5V Reference  typ=uint16  num_adc_bits=12  use_stat=off  use_vardec=off  nam='RTD1_MW'  read_level=1  write_level=1  group='System | I/O Pins | Inputs Config'  use_altref=off  errorHandle=Ignore  errorHandleEdit='Warn'  altref_option_1=off  altref_option_2=off  altref_option_3=off  altref_option_4=off  altref_option_5=off  altref_option_6=off
      settings: SourceProductName=MotoHawk
  motohawk_ain3 : MotoHawk_lib/Analog I//O Blocks/motohawk_ain  res_name='P_Baro'  text_resource=AN11M  code_resource=NONE  val_resource=-1  target=ECU555-48-0403  resource_enum_str=(None)=-1,ECUP=53,DRVP=54,XDRP=55,AN1M=56,AN2M=57,AN3M=58,AN4M=59,AN5M=60,AN9M=64,AN10M=65,AN11M=66,AN14M=69,AN15M=70,AN18M=73,AN19M=74  altref=5V Reference  typ=uint16  num_adc_bits=12  use_stat=off  use_vardec=off  nam='RTD1_MW'  read_level=1  write_level=1  group='System | I/O Pins | Inputs Config'  use_altref=off  errorHandle=Ignore  errorHandleEdit='Warn'  altref_option_1=off  altref_option_2=off  altref_option_3=off  altref_option_4=off  altref_option_5=off  altref_option_6=off
      settings: SourceProductName=MotoHawk
  motohawk_ain4 : MotoHawk_lib/Analog I//O Blocks/motohawk_ain  res_name='U_Bat'  text_resource=AN10M  code_resource=NONE  val_resource=-1  target=ECU555-48-0403  resource_enum_str=(None)=-1,ECUP=53,DRVP=54,XDRP=55,AN1M=56,AN2M=57,AN3M=58,AN4M=59,AN5M=60,AN9M=64,AN10M=65,AN11M=66,AN14M=69,AN15M=70,AN18M=73,AN19M=74  altref=5V Reference  typ=uint16  num_adc_bits=12  use_stat=off  use_vardec=off  nam='RTD1_MW'  read_level=1  write_level=1  group='System | I/O Pins | Inputs Config'  use_altref=off  errorHandle=Ignore  errorHandleEdit='Warn'  altref_option_1=off  altref_option_2=off  altref_option_3=off  altref_option_4=off  altref_option_5=off  altref_option_6=off
      settings: SourceProductName=MotoHawk
  motohawk_ain5 : MotoHawk_lib/Analog I//O Blocks/motohawk_ain  res_name='P_Fuel'  text_resource=AN9M  code_resource=NONE  val_resource=-1  target=ECU555-48-0403  resource_enum_str=(None)=-1,ECUP=53,DRVP=54,XDRP=55,AN1M=56,AN2M=57,AN3M=58,AN4M=59,AN5M=60,AN9M=64,AN10M=65,AN11M=66,AN14M=69,AN15M=70,AN18M=73,AN19M=74  altref=5V Reference  typ=uint16  num_adc_bits=12  use_stat=off  use_vardec=off  nam='RTD1_MW'  read_level=1  write_level=1  group='System | I/O Pins | Inputs Config'  use_altref=off  errorHandle=Ignore  errorHandleEdit='Warn'  altref_option_1=off  altref_option_2=off  altref_option_3=off  altref_option_4=off  altref_option_5=off  altref_option_6=off
      settings: SourceProductName=MotoHawk
  motohawk_ain6 : MotoHawk_lib/Analog I//O Blocks/motohawk_ain  res_name='Load'  text_resource=(None)  code_resource=NONE  val_resource=-1  target=ECU555-48-0403  resource_enum_str=(None)=-1,ECUP=53,DRVP=54,XDRP=55,AN1M=56,AN2M=57,AN3M=58,AN4M=59,AN5M=60,AN9M=64,AN10M=65,AN11M=66,AN14M=69,AN15M=70,AN18M=73,AN19M=74  altref=5V Reference  typ=uint16  num_adc_bits=12  use_stat=off  use_vardec=off  nam='RTD1_MW'  read_level=1  write_level=1  group='System | I/O Pins | Inputs Config'  use_altref=off  errorHandle=Ignore  errorHandleEdit='Warn'  altref_option_1=off  altref_option_2=off  altref_option_3=off  altref_option_4=off  altref_option_5=off  altref_option_6=off
      settings: SourceProductName=MotoHawk
  motohawk_ain7 : MotoHawk_lib/Analog I//O Blocks/motohawk_ain  res_name='IAT'  text_resource=(None)  code_resource=NONE  val_resource=-1  target=ECU555-48-0403  resource_enum_str=(None)=-1,ECUP=53,DRVP=54,XDRP=55,AN1M=56,AN2M=57,AN3M=58,AN4M=59,AN5M=60,AN9M=64,AN10M=65,AN11M=66,AN14M=69,AN15M=70,AN18M=73,AN19M=74  altref=5V Reference  typ=uint16  num_adc_bits=12  use_stat=off  use_vardec=off  nam='RTD1_MW'  read_level=1  write_level=1  group='System | I/O Pins | Inputs Config'  use_altref=off  errorHandle=Ignore  errorHandleEdit='Warn'  altref_option_1=off  altref_option_2=off  altref_option_3=off  altref_option_4=off  altref_option_5=off  altref_option_6=off
      settings: SourceProductName=MotoHawk
  motohawk_ain8 : MotoHawk_lib/Analog I//O Blocks/motohawk_ain  res_name='P_CR'  text_resource=(None)  code_resource=NONE  val_resource=-1  target=ECU555-48-0403  resource_enum_str=(None)=-1,ECUP=53,DRVP=54,XDRP=55,AN1M=56,AN2M=57,AN3M=58,AN4M=59,AN5M=60,AN9M=64,AN10M=65,AN11M=66,AN14M=69,AN15M=70,AN18M=73,AN19M=74  altref=5V Reference  typ=uint16  num_adc_bits=12  use_stat=off  use_vardec=off  nam='RTD1_MW'  read_level=1  write_level=1  group='System | I/O Pins | Inputs Config'  use_altref=off  errorHandle=Ignore  errorHandleEdit='Warn'  altref_option_1=off  altref_option_2=off  altref_option_3=off  altref_option_4=off  altref_option_5=off  altref_option_6=off
      settings: SourceProductName=MotoHawk
  motohawk_callout1 : motohawk_annotations_lib/motohawk_callout1  BlockType_='Mototron_harea'  desc='Read from H/W'  edit_text=Read from H/W  edit_as=0
      settings: SourceProductName=MotoHawk Annotations
  motohawk_callout2 : motohawk_annotations_lib/motohawk_callout1  BlockType_='Mototron_harea'  desc='Convert to Engineering Units'  edit_text=Convert to Engineering Units  edit_as=0
      settings: SourceProductName=MotoHawk Annotations
  motohawk_callout3 : motohawk_annotations_lib/motohawk_callout1  BlockType_='Mototron_harea'  desc='Create a Bus of Sensors'  edit_text=Create a Bus of Sensors  edit_as=0
      settings: SourceProductName=MotoHawk Annotations
  Sensors : Outport  VectorParamsAs1DForOutWhenUnconnected=off
  wires:
  Bus Creator/1 -> Sensors/1
  Engine Speed/1(RPMInst) -> Bus Creator/1  "RPMInst"
  motohawk_ain/1 -> Linear Sensor - MAP/1(ADC)
  motohawk_ain2/1 -> Linear Sensor - T_H2/1(ADC)
  motohawk_ain1/1 -> Linear Sensor - P_H2/1(ADC)
  motohawk_ain3/1 -> Linear Sensor - P_Baro/1(ADC)
  Linear Sensor - P_H2/1(P_H2) -> Bus Creator/4  "P_H2"
  Linear Sensor - T_H2/1(T_H2) -> Bus Creator/5  "T_H2"
  Linear Sensor - P_Baro/1(P_Baro) -> Bus Creator/6  "P_Baro"
  motohawk_ain4/1 -> Linear Sensor - U_Bat/1(ADC)
  Linear Sensor - U_Bat/1(U_Bat) -> Bus Creator/7  "U_Bat"
  motohawk_ain5/1 -> Linear Sensor - P_Fuel/1(ADC)
  Linear Sensor - P_Fuel/1(P_Fuel) -> Bus Creator/8  "P_Fuel"
  motohawk_ain6/1 -> Linear Sensor - Load/1(ADC)
  Linear Sensor - Load/1(Load) -> Bus Creator/9  "Load"
  motohawk_ain7/1 -> Linear Sensor - IAT/1(ADC)
  motohawk_ain8/1 -> Linear Sensor - P_CR/1(ADC)
  Linear Sensor - P_CR/1(P_CR) -> Bus Creator/11  "P_CR"
  Linear Sensor - IAT/1(IAT) -> Switch/3  "IAT"
  Switch/1 -> Bus Creator/10  "IAT"
  In1/1 -> Bus Selector/1
  Bus Creator1/1 -> Bus Creator/12
  Linear Sensor - MAP/1(MAP) -> Switch1/3  "MAP"
  Switch1/1 -> Bus Creator/3  "MAP"
  Bus Selector/1 -> Switch1/1, Switch1/2  "<MAP>"
  Bus Selector/2 -> Switch/1, Switch/2  "<IAT>"
  Bus Selector/3 -> Bus Creator1/1  "<h2 request>"
  Bus Selector/4 -> Bus Creator1/2  "<EGT>"
  Bus Selector/5 -> Bus Creator1/3  "<AFR>"
  Engine Speed/2(RPM) -> Switch2/3  "RPM"
  Switch2/1 -> Bus Creator/2  "RPM"
  Bus Selector/6 -> Switch2/1, Switch2/2  "<RPM>"
